simulink library "n_estimatedLib"  (R2023a)
settings: Solver=VariableStepAuto  StartTime=0.0  StopTime=10.0  RelTol=1e-3
settings Model: Creator=afons  LastModifiedBy=afons

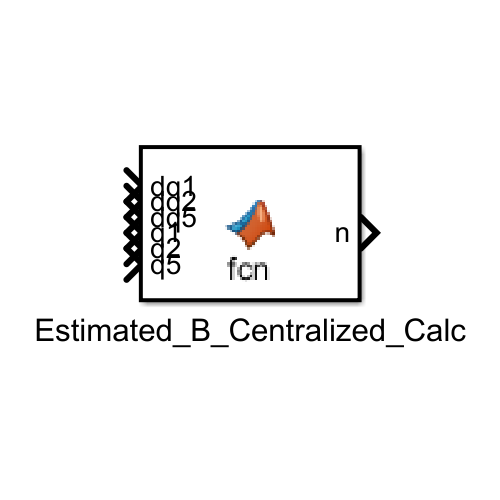
[thumbnail: Simulink's stored preview of the top-level diagram]
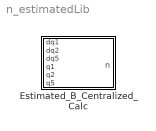
== system n_estimatedLib ==
  Estimated_B_Centralized_Calc : MATLAB Function  TreatAsAtomicUnit=on

== matlab function n_estimatedLib/Estimated_B_Centralized_Calc ==
  data: dq1 input; n output; dq2 input; dq5 input; q1 input; q2 input; q5 input
function n = Estimated_B_Centralized_Calc(dq1,dq2,dq5,q1,q2,q5)
%#codegen

%    This function was generated by the Symbolic Math Toolbox version 9.3.
%    14-Jun-2023 23:35:41

% dq1 = complex(dq1);  % if required to enforce complex operations
% dq2 = complex(dq2);  % if required to enforce complex operations
% dq5 = complex(dq5);  % if required to enforce complex operations
% q1 = complex(q1);  % if required to enforce complex operations
% q2 = complex(q2);  % if required to enforce complex operations
% q5 = complex(q5);  % if required to enforce complex operations
t2 = cos(q1);
t3 = cos(q2);
t4 = sin(q1);
t5 = sin(q2);
t6 = dq1.^2;
t7 = dq2.^2;
t8 = q2.*2.0;
t9 = q5.^2;
t10 = pi./9.0;
t11 = pi.*(2.0./9.0);
t12 = pi.*(2.0./1.5e+1);
t13 = pi.*(4.0./1.5e+1);
t14 = pi./4.5e+1;
t20 = pi.*(1.1e+1./4.5e+1);
t15 = cos(t10);
t16 = cos(t12);
t17 = sin(t10);
t18 = sin(t14);
t19 = -t14;
t21 = q2+t10;
t22 = q2+t12;
t23 = q2+t13;
t25 = q2+t20;
t30 = t8+t11;
t31 = t8+t13;
t39 = t8+t20;
t24 = q2+t19;
t26 = cos(t21);
t27 = sin(t21);
t28 = sin(t22);
t29 = sin(t23);
t33 = cos(t25);
t35 = sin(t25);
t36 = cos(t30);
t37 = sin(t30);
t38 = sin(t31);
t40 = cos(t39);
t41 = sin(t39);
t32 = cos(t24);
t34 = sin(t24);
et1 = t2.*(-2.052933022289608)+t4.*pi.*3.29725e+1-dq1.*dq5.*8.148409067680494e-1+t2.*t16.*1.397925e+1-t2.*t5.*sin(t12).*(9.81e+2./6.4e+1)-t7.*t26.*pi.*1.630057263241001e-1;
et2 = t7.*t27.*pi.*5.285138874693635e-1+dq1.*dq5.*q5.*3.0-dq1.*dq2.*t5.*(5.7e+1./1.6e+2)-dq1.*dq5.*t18.*(3.0./4.0)+dq1.*dq2.*t26.*3.619695120348657e-2;
et3 = dq1.*dq2.*t27.*1.116396458358791e-2+dq1.*dq2.*t28.*6.539669413511747e-2-dq1.*dq2.*t29.*(5.7e+1./1.6e+2)-dq1.*dq5.*t27.*1.255616527394255e-1;
et4 = dq1.*dq2.*t32.*(-2.594522720304148e-1)-dq1.*dq2.*t33.*2.594522720304148e-1-dq1.*dq2.*t34.*8.002099292274005e-2-dq1.*dq2.*t35.*8.002099292274005e-2;
et5 = dq1.*dq2.*t36.*(-1.219907892006508e-1)+dq1.*dq2.*t37.*2.159431252576889e-1+dq1.*dq5.*t34.*(9.0./1.0e+1)-dq1.*dq2.*t38.*(2.97e+2./8.0e+2)+dq1.*dq5.*t35.*(9.0./1.0e+1);
et6 = dq1.*dq5.*t36.*8.148409067680494e-1-dq1.*dq2.*t40.*4.324204533840247e-1+dq1.*dq5.*t37.*2.150524823068501e-1-dq1.*dq2.*t41.*1.333683215379001e-1+dq1.*dq5.*t41.*(3.0./4.0);
et7 = t2.*t3.*t15.*2.616686468573599+t2.*t3.*t16.*(9.81e+2./6.4e+1)-t2.*t3.*t17.*8.484089295394564-t2.*t5.*t15.*8.484089295394564-t2.*t5.*t17.*2.616686468573599;
et8 = t7.*pi.*cos(t22).*(-1.21e+2./1.44e+2)-q5.*t7.*t27.*pi.*(1.1e+1./6.0)-dq1.*dq2.*q5.*t26.*1.255616527394255e-1+dq1.*dq2.*q5.*t32.*(9.0./1.0e+1)+dq1.*dq2.*q5.*t33.*(9.0./1.0e+1)+dq1.*dq2.*q5.*t36.*4.301049646137002e-1-dq1.*dq2.*q5.*t37.*1.629681813536099-dq1.*dq5.*q5.*t36.*3.0+dq1.*dq2.*q5.*t40.*(3.0./2.0)+dq1.*dq2.*t9.*t37.*3.0+q5.*t2.*t3.*t17.*2.943e+1;
et9 = q5.*t2.*t5.*t15.*2.943e+1+dq2.*dq5.*t26.*pi.*(1.1e+1./3.0);
et10 = dq2.*dq5.*(-1.629681813536099)+t5.*t6.*(5.7e+1./3.2e+2)-t4.*t26.*8.484089295394564-t4.*t27.*2.616686468573599-t4.*t28.*(9.81e+2./6.4e+1);
et11 = t6.*t26.*(-1.809847560174329e-2)-t6.*t27.*5.581982291793953e-3-t6.*t28.*3.269834706755874e-2+t6.*t29.*(5.7e+1./3.2e+2);
et12 = t6.*t32.*1.297261360152074e-1+t6.*t33.*1.297261360152074e-1+t6.*t34.*4.001049646137002e-2+t6.*t35.*4.001049646137002e-2;
et13 = t6.*t36.*6.099539460032538e-2-t6.*t37.*1.079715626288445e-1+t6.*t38.*1.85625e-1;
et14 = t6.*t40.*2.162102266920123e-1+t6.*t41.*6.668416076895004e-2+dq2.*dq5.*q5.*6.0-dq2.*dq5.*t18.*(3.0./2.0)+q5.*t4.*t26.*2.943e+1+q5.*t6.*t26.*6.278082636971277e-2-q5.*t6.*t32.*(9.0./2.0e+1)-q5.*t6.*t33.*(9.0./2.0e+1);
et15 = q5.*t6.*t36.*(-2.150524823068501e-1)+q5.*t6.*t37.*8.148409067680494e-1-q5.*t6.*t40.*(3.0./4.0)-t6.*t9.*t37.*(3.0./2.0);
et16 = t6.*4.074204533840247e-1+t7.*8.148409067680494e-1-q5.*t6.*(3.0./2.0)-q5.*t7.*3.0+t6.*t18.*(3.0./8.0)+t7.*t18.*(3.0./4.0)+t4.*t27.*2.943e+1+t6.*t27.*6.278082636971277e-2-t6.*t34.*(9.0./2.0e+1)-t6.*t35.*(9.0./2.0e+1);
et17 = t6.*t36.*(-4.074204533840247e-1)-t6.*t37.*1.075262411534251e-1-t6.*t41.*(3.0./8.0)+q5.*t6.*t36.*(3.0./2.0);
n = [et1+et2+et3+et4+et5+et6+et7+et8+et9;et10+et11+et12+et13+et14+et15;et16+et17];
end
